simulink model "APSA"  (R2014b)
settings: Solver=FixedStepDiscrete  StartTime=0.0  StopTime=180  FixedStep=0.01  RelTol=1e-3
PreLoadFcn:
  | if exist('tl_preloadfcn','file'), tl_preloadfcn(gcs,400); end
PostLoadFcn:
  | if exist('tl_postloadfcn','file'), tl_postloadfcn(gcs,400); end
InitFcn:
  | if exist('tlds_init','file'), tlds_init(gcs); end
StartFcn:
  | if exist('tlds_start','file'), tlds_start(gcs); end
StopFcn:
  | if exist('tlds_stop','file'), tlds_stop(gcs); end
values from neighbouring files (symbols this model uses):
  EERAM_Map_Backward_Values = EERAM_Current_Map_Backward.signals.values(row,:)    [Create_Map.m]    (also in EERAM_Map_Backward_Values_2.mat = [0 0 0 0 0 0 150 150 150 150 150 150 ... (100 elements, 1x10)
  EERAM_Map_Forward_Values = EERAM_Current_Map_Forward.signals.values(row,:)    [Create_Map.m]    (also in EERAM_Map_Forward_Values_2.mat = [150 150 150 150 150 150 150 150 150 150 150 150 ... (100 el)
undefined symbols (not defined in the file or in its folder): sigbuilder_block
libraries: tllib x2
(part 3 of 3)

== stateflow chart APSA/Subsystem/APSA/APSA_chart ==
  state Init [function]
    (default) -> (junction 81) : {Index_vector = 0;
        | Counter_Time = 0;
        | Segments_Cnt = 0;
        | Cnt_Fail_Sens_Current = 0;
        | EERAM_Current_Map_Forward_Write = EERAM_Current_Map_Forward_Read;
        | EERAM_Current_Map_Backward_Write = EERAM_Current_Map_Backward_Read;}
  state Check_Min_Threshold [function]
    (default) -> (junction 206)
    (junction 206) -> (junction 207) [order 2] : [ Cnt_Fail_Sens_Current != 0 ]
    (junction 206) -> (junction 205) [order 1] : [ Current <=  MIN_CURRENT_THRESHOLD ]
    (junction 205) -> (junction 209) [order 1] : [ Cnt_Fail_Sens_Current > MAX_CNT_MIN_CURRENT_THRESHOLD ]
    (junction 207) -> (junction 211) : { Cnt_Fail_Sens_Current--; }
    (junction 206) -> (junction 208) [order 3] : { Fail_Sens_Current = APSA_FALSE;}
    (junction 205) -> (junction 210) [order 2] : { Cnt_Fail_Sens_Current++; }
    (junction 209) -> (junction 212) : { Fail_Sens_Current = APSA_TRUE; }
    (junction 211) -> (junction 208)
    (junction 210) -> (junction 208)
    (junction 212) -> (junction 210)
    (junction 208) -> (junction 213)
  state SetTimer_Delay [function]
    (default) -> (junction 1476)
    (junction 1476) -> (junction 1477) [order 1] : [APSA_Delay >1]
        | {APSA_Delay --;}
    (junction 1476) -> (junction 1478) [order 2]
    (junction 1477) -> (junction 1479)
    (junction 1478) -> (junction 1479)
  state Calculate_Lenght_Segment [function]
    (default) -> (junction 360) : {Mod=(Lenght_Motor_Stroke)%%MAX_NUM_ELEMENT;}
    (junction 360) -> (junction 361) [order 1] : [Mod == 0]
    (junction 360) -> (junction 371) [order 2] : {Lenght_Segment=((Lenght_Motor_Stroke/MAX_NUM_ELEMENT)+1);}
    (junction 361) -> (junction 365) : {Lenght_Segment = Lenght_Motor_Stroke/MAX_NUM_ELEMENT;}
    (junction 365) -> (junction 371)
    (junction 371) -> (junction 374)
  state ANTIPINCH_ACTIVE_FORWARD
    en:
    Counter_Time = 0;
    //ex: EERAM_Current_Map_Forward_Write = EERAM_Current_Map_Forward_Write - (Average_Difference);
    state WAIT_INRUSH_TIME_FORWARD
      WAIT_INRUSH_TIME_FORWARD -> (junction 87) [order 1]
      (junction 87) -> (junction 88) [order 1] : [Counter_Time < INRUSH_TIME]
          | {Counter_Time ++;}
      (junction 87) -> (junction 90) [order 2]
      (junction 88) -> (junction 93)
      (junction 93) -> (junction 797) [order 1] : [Counter_Time == INRUSH_TIME -1]
          | {Reset_Filter = 1;}
      (junction 93) -> (junction 795) [order 2] : {Reset_Filter = 0;}
      (junction 797) -> (junction 799)
      (junction 795) -> (junction 90)
      (junction 799) -> (junction 795)
      (junction 90) -> (junction 96)
      (junction 96) -> (junction 832) [order 1] : [Current_Peak <= Current]
          | {Current_Peak = Current;}
      (junction 96) -> (junction 830) [order 2]
      (junction 832) -> (junction 834)
      (junction 834) -> (junction 830)
    state Antipinch_Active
    state WAIT_ADAPTATION_TIME_FORWARD
      en:
      Average_Current = 0;
      Average_EERAM_Current_Map = 0;
      Average_Difference = 0;
      Segments_Cnt = 0;
      Index_vector = Hall_Counter_Forward / Lenght_Segment;
      WAIT_ADAPTATION_TIME_FORWARD -> (junction 99) [order 1]
      (junction 99) -> (junction 100) [order 1] : [Counter_Time < ADAPTATION_TIME]
          | {Counter_Time++;
          | Average_Current += Current;}
      (junction 99) -> (junction 101) [order 2]
      (junction 100) -> (junction 127)
      (junction 127) -> (junction 128) [order 1] : [Hall_Counter_Forward >= ((Index_vector * Lenght_Segment) + Lenght_Segment) ...
          | && (Index_vector <= (MAX_NUM_ELEMENT-1))]
      (junction 127) -> (junction 102) [order 2]
      (junction 128) -> (junction 130) : {//Average_Current += Current;
          | //EERAM_Current_Map_Forward_Write[Index_vector] = Map_Realignment(EERAM_Current_Map_Forward_Read[Index_vector],EERAM_Threshold_Attention_Higher);
          | Average_EERAM_Current_Map += EERAM_Current_Map_Forward_Read[Index_vector];
          | Index_vector++;
          | Segments_Cnt++;}
      (junction 102) -> (junction 101)
      (junction 130) -> (junction 102)
    state CHECK_ANTIPINCH_FORWARD
      en:
      cnt_antipinch = 0;
      Index_vector = Hall_Counter_Forward / Lenght_Segment;
      Current_Read = Current;
      Counter_Sample_Current = 1;
      APSA_Delay = 0;
      Cmd_Motor_Lift_Old = Cmd_Motor_Lift;
      state CounterManagerUpFwd(ResetCounter) [function]
        (default) -> (junction 1125) : {BitMaskIndex = (Index_vector / 8) ;
            | BitPosition = Index_vector - (BitMaskIndex * 8);
            | BitPosition = ((8 - BitPosition)*2 ) -2  ;}
        (junction 1125) -> (junction 1127) [order 1] : [ResetCounter == APSA_TRUE]
            | {CounterVectorUpFwd_Write[BitMaskIndex] = 0;
            | CounterVectorUpFwd_Write[BitMaskIndex] = 0;}
        (junction 1125) -> (junction 1083) [order 2]
        (junction 1127) -> (junction 1082)
        (junction 1083) -> (junction 1082) [commented out] : /*Counter = 4*/
            | [((CounterVectorFwd[BitMaskIndex] & (COUNT_BIT_TWO << (BitPosition))) ==  COUNT_BIT_TWO  << (BitPosition) ) ...
            | && ((CounterVectorFwd[BitMaskIndex] & (COUNT_BIT_ONE << (BitPosition))) ==  COUNT_BIT_ONE  << (BitPosition) )]
            | {CounterVectorFwd[BitMaskIndex] = (CounterVectorFwd[BitMaskIndex] & ~(COUNT_BIT_ONE << (BitPosition) ));
            | CounterVectorFwd[BitMaskIndex] = (CounterVectorFwd[BitMaskIndex] & ~(COUNT_BIT_TWO << (BitPosition)) );}
        (junction 1082) -> (junction 1085)
        (junction 1083) -> (junction 1084)
        (junction 1084) -> (junction 1085) [order 1] : [((CounterVectorUpFwd_Read[BitMaskIndex] & ((COUNT_BIT_TWO << (BitPosition)))) ==  COUNT_BIT_TWO  << (BitPosition) )]
            | /*{CounterVectorUpFwd_Write[BitMaskIndex] = (CounterVectorUpFwd_Read[BitMaskIndex] | COUNT_BIT_TWO << (BitPosition) );
            | CounterVectorUpFwd_Write[BitMaskIndex] = (CounterVectorUpFwd_Read[BitMaskIndex] | COUNT_BIT_ONE << (BitPosition) );}*/
            | {CounterVectorUpFwd_Write[BitMaskIndex] = (CounterVectorUpFwd_Read[BitMaskIndex] & ~(COUNT_BIT_ONE << (BitPosition) ));
            | CounterVectorUpFwd_Write[BitMaskIndex] = (CounterVectorUpFwd_Read[BitMaskIndex] & ~(COUNT_BIT_TWO << (BitPosition)) );
            | UpdateTrh = APSA_TRUE;}
        (junction 1084) -> (junction 1086) [order 2]
        (junction 1085) -> (junction 1087)
        (junction 1086) -> (junction 1087) [order 1] : [(CounterVectorUpFwd_Read[BitMaskIndex] & (COUNT_BIT_ONE << (BitPosition)))  == (COUNT_BIT_ONE << (BitPosition))  ]
            | {CounterVectorUpFwd_Write[BitMaskIndex] = (CounterVectorUpFwd_Read[BitMaskIndex] & ~(COUNT_BIT_ONE << (BitPosition)));
            | CounterVectorUpFwd_Write[BitMaskIndex] = (CounterVectorUpFwd_Read[BitMaskIndex] | (COUNT_BIT_TWO << (BitPosition)));}
        (junction 1087) -> (junction 1089)
        (junction 1086) -> (junction 1088) [order 2]
        (junction 1088) -> (junction 1089) : /*[(CounterVectorFwd[BitMaskIndex]  & (COUNT_BIT_ONE << ( BitPosition))) != (COUNT_BIT_ONE << BitPosition)]*/
            | {CounterVectorUpFwd_Write[BitMaskIndex] = (CounterVectorUpFwd_Read[BitMaskIndex] | (COUNT_BIT_ONE << (BitPosition) ));}
        (junction 1088) -> (junction 1090) [commented out]
        (junction 1089) -> (junction 1091) [commented out]
        (junction 1090) -> (junction 1091) [commented out] : {CounterVectorFwd[BitMaskIndex] = (CounterVectorFwd[BitMaskIndex] & ~COUNT_BIT_ONE << (BitPosition) );
            | CounterVectorFwd[BitMaskIndex] = (CounterVectorFwd[BitMaskIndex] & ~COUNT_BIT_TWO << (BitPosition) );}
      state CounterManagerDownFwd(ResetCounter) [function]
        (default) -> (junction 1133) : {BitMaskIndex = Index_vector / 8;
            | BitPosition = Index_vector - (BitMaskIndex * 8);
            | BitPosition = ((8 - BitPosition)*2 ) -2  ;}
        (junction 1133) -> (junction 1134) [order 1] : [ResetCounter == APSA_TRUE]
            | {CounterVectorDownFwd_Write[BitMaskIndex] = 0;
            | CounterVectorDownFwd_Write[BitMaskIndex] = 0;}
        (junction 1133) -> (junction 1136) [order 2]
        (junction 1134) -> (junction 1135)
        (junction 1136) -> (junction 1135) [commented out] : /*Counter = 4*/
            | [((CounterVectorFwd[BitMaskIndex] & (COUNT_BIT_TWO << (BitPosition))) ==  COUNT_BIT_TWO  << (BitPosition) ) ...
            | && ((CounterVectorFwd[BitMaskIndex] & (COUNT_BIT_ONE << (BitPosition))) ==  COUNT_BIT_ONE  << (BitPosition) )]
            | {CounterVectorFwd[BitMaskIndex] = (CounterVectorFwd[BitMaskIndex] & ~(COUNT_BIT_ONE << (BitPosition) ));
            | CounterVectorFwd[BitMaskIndex] = (CounterVectorFwd[BitMaskIndex] & ~(COUNT_BIT_TWO << (BitPosition)) );}
        (junction 1135) -> (junction 1138)
        (junction 1136) -> (junction 1137)
        (junction 1137) -> (junction 1138) [order 1] : [((CounterVectorDownFwd_Read[BitMaskIndex] & ((COUNT_BIT_TWO << (BitPosition)))) ==  COUNT_BIT_TWO  << (BitPosition) )]
            | /*{CounterVectorDownFwd_Write[BitMaskIndex] = (CounterVectorFwd_Read[BitMaskIndex] | COUNT_BIT_TWO << (BitPosition) );
            | CounterVectorDownFwd_Write[BitMaskIndex] = (CounterVectorFwd_Read[BitMaskIndex] | COUNT_BIT_ONE << (BitPosition) );}*/
            | {CounterVectorDownFwd_Write[BitMaskIndex] = (CounterVectorDownFwd_Read[BitMaskIndex] & ~(COUNT_BIT_ONE << (BitPosition) ));
            | CounterVectorDownFwd_Write[BitMaskIndex] = (CounterVectorDownFwd_Read[BitMaskIndex] & ~(COUNT_BIT_TWO << (BitPosition)) );
            | UpdateTrh = APSA_TRUE;}
        (junction 1137) -> (junction 1139) [order 2]
        (junction 1138) -> (junction 1140)
        (junction 1139) -> (junction 1140) [order 1] : [(CounterVectorDownFwd_Read[BitMaskIndex] & (COUNT_BIT_ONE << (BitPosition)))  == (COUNT_BIT_ONE << (BitPosition))  ]
            | {CounterVectorDownFwd_Write[BitMaskIndex] = (CounterVectorDownFwd_Read[BitMaskIndex] & ~(COUNT_BIT_ONE << (BitPosition)));
            | CounterVectorDownFwd_Write[BitMaskIndex] = (CounterVectorDownFwd_Read[BitMaskIndex] | (COUNT_BIT_TWO << (BitPosition)));}
        (junction 1140) -> (junction 1142)
        (junction 1139) -> (junction 1141) [order 2]
        (junction 1141) -> (junction 1142) : /*[(CounterVectorFwd[BitMaskIndex]  & (COUNT_BIT_ONE << ( BitPosition))) != (COUNT_BIT_ONE << BitPosition)]*/
            | {CounterVectorDownFwd_Write[BitMaskIndex] = (CounterVectorDownFwd_Read[BitMaskIndex] | (COUNT_BIT_ONE << (BitPosition) ));}
        (junction 1141) -> (junction 1143) [commented out]
        (junction 1142) -> (junction 1144) [commented out]
        (junction 1143) -> (junction 1144) [commented out] : {CounterVectorFwd[BitMaskIndex] = (CounterVectorFwd[BitMaskIndex] & ~COUNT_BIT_ONE << (BitPosition) );
            | CounterVectorFwd[BitMaskIndex] = (CounterVectorFwd[BitMaskIndex] & ~COUNT_BIT_TWO << (BitPosition) );}
      CHECK_ANTIPINCH_FORWARD -> (junction 275) [order 1] : {SetTimer_Delay();}
      (junction 275) -> (junction 891) [order 2]
      (junction 891) -> (junction 1491) [order 1] : [ Hall_Counter_Forward >= ((Index_vector * Lenght_Segment) + Lenght_Segment) ...
          | && (Index_vector < (MAX_NUM_ELEMENT - 1))]
      (junction 1491) -> (junction 1488) [order 2]
      (junction 1488) -> (junction 1497) [order 1] : /* with voltage drop  || stop lift motor inhibit antipinch for DROP_DELAY */
          | [(((Vbatt_Old - Vbatt) >= VBATT_DROP) || ((Vbatt - Vbatt_Old) >= VBATT_DROP)) ...
          | || ((Cmd_Motor_Lift == APSA_CMD_STOP) && ((Cmd_Motor_Lift_Old == APSA_CMD_FORWARD) || (Cmd_Motor_Lift_Old == APSA_CMD_BACKWARD)))]
          | {APSA_Delay = DROP_DELAY;}
      (junction 275) -> (junction 706) [order 1] : [cnt_antipinch >T_ANTIPINCH]
      (junction 891) -> (junction 282) [order 2] : {Current_Read += Current;
          | Counter_Sample_Current ++;}
      (junction 1491) -> (junction 1500) [order 1] : /*this check is used to avoid currentread saturation
          | during drop delay*/
          | [APSA_Delay > 1]
      (junction 1488) -> (junction 1494) [order 2] : {Current_Read_Average = Current_Read / Counter_Sample_Current;
          |  Delta_Current_actual = ( Current_Read_Average - (EERAM_Current_Map_Forward_Read[Index_vector] + Average_Difference ) - Delta_Current_previuos );}
      (junction 1497) -> (junction 1496)
      (junction 1494) -> (junction 1496) [order 1] : [APSA_Delay ==  1]
          | {Delta_Current_previuos  += Delta_Current_actual;
          | APSA_Delay = 0; }
      (junction 1494) -> (junction 280) [order 2]
      (junction 1496) -> (junction 1108)
      (junction 280) -> (junction 883) [order 2] : {cnt_antipinch = 0;
          | UpdateTrh = APSA_FALSE;}
      (junction 280) -> (junction 329) [order 1] : [(Delta_Current_actual  > Threshold_AntiPinch_Update) ...
          | && (cnt_antipinch < T_ANTIPINCH)  ]
          | {cnt_antipinch++; }
      (junction 883) -> (junction 299) : /*CHECK_ATTENTION_THRESHOLD*/
      (junction 299) -> (junction 302) [order 1] : /*UPPER_THRESHOLD*/
          | [Delta_Current_actual > Threshold_Attention_Update ]
          | {CounterManagerUpFwd(APSA_FALSE);
          | Delta_Current_previuos  += Threshold_Attention_Update;}
      (junction 302) -> (junction 1108) [order 1] : [UpdateTrh == APSA_TRUE]
          | {EERAM_Current_Map_Forward_Write[Index_vector] += (Delta_Current_actual / DELTA_1);}
      (junction 299) -> (junction 304) [order 2] : /*Reset counter Up*/
          | {CounterManagerUpFwd(APSA_TRUE); }
      (junction 302) -> (junction 1109) [order 2]
      (junction 1108) -> (junction 1299)
      (junction 1109) -> (junction 1299)
      (junction 1299) -> (junction 1106)
      (junction 304) -> (junction 306) [order 1] : /*LOWER_THRESHOLD*/
          | [Delta_Current_actual < (-Threshold_Attention_Update) ...
          | && EERAM_Current_Map_Forward_Read[Index_vector] > MIN_CURRENT_THRESHOLD ]
          | {CounterManagerDownFwd(APSA_FALSE);
          | Delta_Current_previuos  += Delta_Current_actual;}
      (junction 306) -> (junction 1106) [order 1] : [UpdateTrh == APSA_TRUE]
          | {EERAM_Current_Map_Forward_Write[Index_vector]-= (-Delta_Current_actual / DELTA_2 );}
      (junction 329) -> (junction 331) [order 1] : [cnt_antipinch >= T_ANTIPINCH]
          | {Antipinch_Active = APSA_ACTIVE;}
      (junction 304) -> (junction 885) [order 2] : /*Reset counter Down*/
          | {CounterManagerDownFwd(APSA_TRUE);
          | Delta_Current_previuos  += Delta_Current_actual;}
      (junction 306) -> (junction 887) [order 2]
      (junction 1106) -> (junction 1115)
      (junction 329) -> (junction 333) [order 2]
      (junction 331) -> (junction 335)
      (junction 1500) -> (junction 333)
      (junction 335) -> (junction 333)
      (junction 885) -> (junction 335)
      (junction 887) -> (junction 885)
      (junction 1115) -> (junction 887)
      (junction 333) -> (junction 338) : {Check_Min_Threshold();
          | Index_vector++;
          | Current_Read = Current;
          | Counter_Sample_Current = 1;
          | Vbatt_Old = Vbatt;
          | Cmd_Motor_Lift_Old = Cmd_Motor_Lift; }
      (junction 706) -> (junction 282)
      (junction 282) -> (junction 338)
      (junction 338) -> (junction 346)
    (default) -> WAIT_INRUSH_TIME_FORWARD : {Current_Peak = Current;}
    WAIT_INRUSH_TIME_FORWARD -> (junction 875) [order 1] : [Counter_Time >= INRUSH_TIME]
        | {Counter_Time = 0;}
    (junction 875) -> ANTIPINCH_ACTIVE_FORWARD.Antipinch_Active [commented out] : [Current  > (Current_Peak - DELTA_PEACK)]
        | {Antipinch_Active = APSA_ACTIVE;}
    (junction 875) -> WAIT_ADAPTATION_TIME_FORWARD
    (junction 857) -> ANTIPINCH_ACTIVE_FORWARD.Antipinch_Active
    WAIT_ADAPTATION_TIME_FORWARD -> CHECK_ANTIPINCH_FORWARD [order 1] : [Counter_Time >= ADAPTATION_TIME]
        | {Average_Current /= Counter_Time;
        | Average_EERAM_Current_Map /= Segments_Cnt;
        | Average_Difference  = Average_Current - Average_EERAM_Current_Map ;
        | //EERAM_Current_Map_Forward_Write = EERAM_Current_Map_Forward_Write + (Average_Difference);
        | Delta_Current_previuos = 0;
        | Threshold_Attention_Update = EERAM_Threshold_Antipinch_Forward / 2;
        | Threshold_AntiPinch_Update = EERAM_Threshold_Antipinch_Forward ;}
    CHECK_ANTIPINCH_FORWARD -> (junction 857) [order 1] : [Antipinch_Active == APSA_ACTIVE]
        | {Current_Read_Average = 0;}
  state IDLE
    en:
    Antipinch_Active = APSA_NOT_ACTIVE;
  state WRITE_MAP_FORWARD
    en:
    Index_vector = Hall_Counter_Forward / Lenght_Segment;
    //Current_Read = Current;
    Current_Read = 0;
    Counter_Sample_Current = 1;
    Index_peak_time = 0;
    Counter_Time = 0;
    WRITE_MAP_FORWARD -> (junction 1371) [order 1]
    (junction 1371) -> (junction 1368) [order 1] : [Counter_Time < PEAK_FILTER_TIME]
        | {Counter_Time++;}
    (junction 1368) -> (junction 1366) [order 1] : [Hall_Counter_Forward >= ((Index_vector * Lenght_Segment) + Lenght_Segment) ...
        | && (Index_vector <= (MAX_NUM_ELEMENT-1))]
        | {Index_vector++;}
    (junction 1371) -> (junction 1369) [order 2] : //[Counter_Time >= PEAK_FILTER_TIME]
    (junction 1368) -> (junction 1366) [order 2]
    (junction 1366) -> (junction 1381)
    (junction 1381) -> (junction 1383)
    (junction 1369) -> (junction 1370) [order 1] : /*Thi for cycle is used to erase the hit of the current */
        | [Index_peak_time <= Index_vector]
    (junction 1370) -> (junction 1367) : {EERAM_Current_Map_Forward_Write[Index_peak_time] = Current;
        | Index_peak_time ++;}
    (junction 1367) -> (junction 1369)
    (junction 1369) -> (junction 1392) [order 2]
    (junction 1392) -> (junction 63) [order 2]
    (junction 1392) -> (junction 63) [order 1] : [Current_Read == 0]
        | {Current_Read = Current;}
    (junction 63) -> (junction 64) [order 1] : [Hall_Counter_Forward >= ((Index_vector * Lenght_Segment) + Lenght_Segment) ...
        | && (Index_vector <= (MAX_NUM_ELEMENT-1))]
    (junction 64) -> (junction 730) [order 1] : [Counter_Sample_Current == 0 ...
        | || Current_Read == 0 ]
    (junction 63) -> (junction 66) [order 2] : {Current_Read += Current;
        | Counter_Sample_Current++;}
    (junction 64) -> (junction 734) [order 2] : {Current_Read_Average = Current_Read / Counter_Sample_Current;}
    (junction 730) -> (junction 732) : {Current_Read_Average = Current;}
    (junction 732) -> (junction 734)
    (junction 734) -> (junction 66) : {EERAM_Current_Map_Forward_Write[Index_vector] = Current_Read_Average;
        | Check_Min_Threshold();
        | Current_Read=Current;
        | Counter_Sample_Current = 1;
        | Index_vector++;}
    (junction 66) -> (junction 717)
    (junction 1383) -> (junction 717)
  state WRITE_MAP_BACKWARD
    en:
    Index_vector = Hall_Counter_Backward / Lenght_Segment;
    // Current_Read = Current;
    Current_Read = 0;
    Counter_Sample_Current = 1;
    Counter_Time = 0;
    Index_peak_time = 0;
    WRITE_MAP_BACKWARD -> (junction 1342) [order 1]
    (junction 1342) -> (junction 1340) [order 1] : [Counter_Time < PEAK_FILTER_TIME]
        | {Counter_Time++;}
    (junction 1340) -> (junction 1343) [order 1] : [ (Hall_Counter_Backward >= ((Index_vector * Lenght_Segment) + Lenght_Segment)) ...
        | && (Index_vector <= (MAX_NUM_ELEMENT-1))]
        | {Index_vector++;}
    (junction 1340) -> (junction 1343) [order 2]
    (junction 1342) -> (junction 1322) [order 2] : //[Counter_Time >= PEAK_FILTER_TIME]
    (junction 1343) -> (junction 1386)
    (junction 1386) -> (junction 1388)
    (junction 1322) -> (junction 1325) [order 1] : [Index_peak_time <= Index_vector]
    (junction 1325) -> (junction 1326) : {EERAM_Current_Map_Backward_Write[Index_peak_time] = Current;
        | Index_peak_time ++;}
    (junction 1326) -> (junction 1322)
    (junction 1322) -> (junction 1397) [order 2]
    (junction 1397) -> (junction 633) [order 2]
    (junction 1397) -> (junction 633) [order 1] : [Current_Read == 0]
        | {Current_Read = Current;}
    (junction 633) -> (junction 639) [order 1] : [ (Hall_Counter_Backward >= ((Index_vector * Lenght_Segment) + Lenght_Segment)) ...
        | && (Index_vector <= (MAX_NUM_ELEMENT-1))]
    (junction 639) -> (junction 739) [order 1] : [Counter_Sample_Current == 0 ...
        | || Current_Read == 0 ]
    (junction 633) -> (junction 632) [order 2] : {Current_Read += Current;
        | Counter_Sample_Current++;}
    (junction 639) -> (junction 641) [order 2] : {Current_Read_Average = Current_Read / Counter_Sample_Current;}
    (junction 739) -> (junction 741) : {Current_Read_Average =Current;}
    (junction 641) -> (junction 632) : {EERAM_Current_Map_Backward_Write[Index_vector]=Current_Read_Average;
        | Check_Min_Threshold();
        | Current_Read = Current;
        | Counter_Sample_Current = 1;
        | Index_vector++;}
    (junction 741) -> (junction 641)
    (junction 632) -> (junction 635)
    (junction 1388) -> (junction 635)
  state ANTIPINCH_ACTIVE_BACKWARD
    en:
    Counter_Time = 0;
    //ex: EERAM_Current_Map_Backward_Write = EERAM_Current_Map_Backward_Write - (Average_Difference);
    state WAIT_INRUSH_TIME_BACKWARD
      WAIT_INRUSH_TIME_BACKWARD -> (junction 803) [order 1]
      (junction 803) -> (junction 804) [order 1] : [Counter_Time < INRUSH_TIME]
          | {Counter_Time ++;}
      (junction 803) -> (junction 811) [order 2]
      (junction 804) -> (junction 807)
      (junction 807) -> (junction 817) [order 1] : [Counter_Time == INRUSH_TIME -1]
          | {Reset_Filter = 1;}
      (junction 807) -> (junction 813) [order 2] : {Reset_Filter = 0;}
      (junction 817) -> (junction 814)
      (junction 813) -> (junction 811)
      (junction 814) -> (junction 813)
      (junction 811) -> (junction 866)
      (junction 866) -> (junction 870) [order 1] : [Current_Peak <= Current]
          | {Current_Peak = Current;}
      (junction 866) -> (junction 869) [order 2]
      (junction 870) -> (junction 872)
      (junction 872) -> (junction 869)
    state Antipinch_Active
    state WAIT_ADAPTATION_TIME_BACKWARD
      en:
      Average_Current = 0;
      Average_EERAM_Current_Map = 0;
      Average_Difference = 0;
      Segments_Cnt = 0;
      Index_vector=Hall_Counter_Backward/Lenght_Segment;
      WAIT_ADAPTATION_TIME_BACKWARD -> (junction 656) [order 1]
      (junction 656) -> (junction 651) [order 1] : [Counter_Time < ADAPTATION_TIME]
          | {Counter_Time++;
          | Average_Current += Current;}
      (junction 656) -> (junction 652) [order 2]
      (junction 651) -> (junction 645)
      (junction 645) -> (junction 647) [order 1] : [Hall_Counter_Backward >= ((Index_vector * Lenght_Segment) + Lenght_Segment) ...
          | && (Index_vector <= (MAX_NUM_ELEMENT - 1))]
      (junction 645) -> (junction 654) [order 2]
      (junction 647) -> (junction 655) : {//Current_Read_Average = Current;
          | //Current_Read_Average = Current_Read / Counter_Sample_Current;
          | //Average_Current += Current_Read_Average;
          | //EERAM_Current_Map_Backward_Write[Index_vector]=Map_Realignment(EERAM_Current_Map_Backward_Read[Index_vector],EERAM_Threshold_Attention_Lower);
          | Average_EERAM_Current_Map += EERAM_Current_Map_Backward_Read[Index_vector];
          | Index_vector++;
          | Segments_Cnt++;}
      (junction 654) -> (junction 652)
      (junction 655) -> (junction 654)
    state CHECK_ANTIPINCH_BACKWARD
      en:
      cnt_antipinch = 0;
      Index_vector = Hall_Counter_Backward / Lenght_Segment;
      Current_Read = Current;
      Counter_Sample_Current = 1;
      Vbatt_Old = Vbatt;
      APSA_Delay = 0;
      Cmd_Motor_Lift_Old = Cmd_Motor_Lift;
      state CounterManagerDownBwd(ResetCounter) [function]
        (default) -> (junction 1257) : {BitMaskIndex = Index_vector / 8;
            | BitPosition = Index_vector - (BitMaskIndex * 8);
            | BitPosition = ((8 - BitPosition)*2 ) -2  ;}
        (junction 1257) -> (junction 1258) [order 1] : [ResetCounter == APSA_TRUE]
            | {CounterVectorDownBwd_Write[BitMaskIndex] = 0;
            | CounterVectorDownBwd_Write[BitMaskIndex] = 0;}
        (junction 1257) -> (junction 1260) [order 2]
        (junction 1258) -> (junction 1259)
        (junction 1260) -> (junction 1259) [commented out] : /*Counter = 4*/
            | [((CounterVectorBwd[BitMaskIndex] & (COUNT_BIT_TWO << (BitPosition))) ==  COUNT_BIT_TWO  << (BitPosition) ) ...
            | && ((CounterVectorBwd[BitMaskIndex] & (COUNT_BIT_ONE << (BitPosition))) ==  COUNT_BIT_ONE  << (BitPosition) )]
            | {CounterVectorBwd[BitMaskIndex] = (CounterVectorBwd[BitMaskIndex] & ~(COUNT_BIT_ONE << (BitPosition) ));
            | CounterVectorBwd[BitMaskIndex] = (CounterVectorBwd[BitMaskIndex] & ~(COUNT_BIT_TWO << (BitPosition)) );}
        (junction 1259) -> (junction 1262)
        (junction 1260) -> (junction 1261)
        (junction 1261) -> (junction 1262) [order 1] : /*Counter = 3*/
            | [((CounterVectorDownBwd_Read[BitMaskIndex] & ((COUNT_BIT_TWO << (BitPosition)))) ==  COUNT_BIT_TWO  << (BitPosition) )]
            | /*{CounterVectorBwd[BitMaskIndex] = (CounterVectorBwd[BitMaskIndex] | COUNT_BIT_TWO << (BitPosition) );
            | CounterVectorBwd[BitMaskIndex] = (CounterVectorBwd[BitMaskIndex] | COUNT_BIT_ONE << (BitPosition) );}*/
            | {CounterVectorDownBwd_Write[BitMaskIndex] = (CounterVectorDownBwd_Read[BitMaskIndex] & ~(COUNT_BIT_ONE << (BitPosition) ));
            | CounterVectorDownBwd_Write[BitMaskIndex] = (CounterVectorDownBwd_Read[BitMaskIndex] & ~(COUNT_BIT_TWO << (BitPosition)) );
            | UpdateTrh = APSA_TRUE;}
        (junction 1261) -> (junction 1263) [order 2]
        (junction 1262) -> (junction 1264)
        (junction 1263) -> (junction 1264) [order 1] : /*Counter = 2*/
            | [(CounterVectorDownBwd_Read[BitMaskIndex] & (COUNT_BIT_ONE << (BitPosition)))  == (COUNT_BIT_ONE << (BitPosition))]
            | {CounterVectorDownBwd_Write[BitMaskIndex] = (CounterVectorDownBwd_Read[BitMaskIndex] & ~(COUNT_BIT_ONE << (BitPosition)));
            | CounterVectorDownBwd_Write[BitMaskIndex] = (CounterVectorDownBwd_Read[BitMaskIndex] | (COUNT_BIT_TWO << (BitPosition)));}
        (junction 1263) -> (junction 1265) [order 2]
        (junction 1264) -> (junction 1266)
        (junction 1265) -> (junction 1266) : /*Counter = 1*/
            | //[(CounterVectorBwd_Read[BitMaskIndex]  & (COUNT_BIT_ONE << ( BitPosition))) != (COUNT_BIT_ONE << BitPosition)]
            | {CounterVectorDownBwd_Write[BitMaskIndex] = (CounterVectorDownBwd_Read[BitMaskIndex] | (COUNT_BIT_ONE << (BitPosition) ));}
        (junction 1265) -> (junction 1267) [commented out]
        (junction 1266) -> (junction 1268) [commented out]
        (junction 1267) -> (junction 1268) [commented out] : {CounterVectorBwd[BitMaskIndex] = (CounterVectorBwd[BitMaskIndex] & ~COUNT_BIT_ONE << (BitPosition) );
            | CounterVectorBwd[BitMaskIndex] = (CounterVectorBwd[BitMaskIndex] & ~COUNT_BIT_TWO << (BitPosition) );}
      state CounterManagerUpBwd(ResetCounter) [function]
        (default) -> (junction 1249) : {BitMaskIndex = Index_vector / 8;
            | BitPosition = Index_vector - (BitMaskIndex * 8);
            | BitPosition = ((8 - BitPosition)*2 ) -2  ;}
        (junction 1249) -> (junction 1251) [order 1] : [ResetCounter == APSA_TRUE]
            | {CounterVectorUpBwd_Write[BitMaskIndex] = 0;
            | CounterVectorUpBwd_Write[BitMaskIndex] = 0;}
        (junction 1251) -> (junction 1039)
        (junction 1249) -> (junction 1042) [order 2]
        (junction 1042) -> (junction 1039) [commented out] : /*Counter = 4*/
            | [((CounterVectorBwd[BitMaskIndex] & (COUNT_BIT_TWO << (BitPosition))) ==  COUNT_BIT_TWO  << (BitPosition) ) ...
            | && ((CounterVectorBwd[BitMaskIndex] & (COUNT_BIT_ONE << (BitPosition))) ==  COUNT_BIT_ONE  << (BitPosition) )]
            | {CounterVectorBwd[BitMaskIndex] = (CounterVectorBwd[BitMaskIndex] & ~(COUNT_BIT_ONE << (BitPosition) ));
            | CounterVectorBwd[BitMaskIndex] = (CounterVectorBwd[BitMaskIndex] & ~(COUNT_BIT_TWO << (BitPosition)) );}
        (junction 1039) -> (junction 1032)
        (junction 1042) -> (junction 1037)
        (junction 1037) -> (junction 1032) [order 1] : /*Counter = 3*/
            | [((CounterVectorUpBwd_Read[BitMaskIndex] & ((COUNT_BIT_TWO << (BitPosition)))) ==  COUNT_BIT_TWO  << (BitPosition) )]
            | /*{CounterVectorBwd[BitMaskIndex] = (CounterVectorBwd[BitMaskIndex] | COUNT_BIT_TWO << (BitPosition) );
            | CounterVectorBwd[BitMaskIndex] = (CounterVectorBwd[BitMaskIndex] | COUNT_BIT_ONE << (BitPosition) );}*/
            | {CounterVectorUpBwd_Write[BitMaskIndex] = (CounterVectorUpBwd_Read[BitMaskIndex] & ~(COUNT_BIT_ONE << (BitPosition) ));
            | CounterVectorUpBwd_Write[BitMaskIndex] = (CounterVectorUpBwd_Read[BitMaskIndex] & ~(COUNT_BIT_TWO << (BitPosition)) );
            | UpdateTrh = APSA_TRUE;}
        (junction 1037) -> (junction 1036) [order 2]
        (junction 1032) -> (junction 1033)
        (junction 1036) -> (junction 1033) [order 1] : /*Counter = 2*/
            | [(CounterVectorUpBwd_Read[BitMaskIndex] & (COUNT_BIT_ONE << (BitPosition)))  == (COUNT_BIT_ONE << (BitPosition))]
            | {CounterVectorUpBwd_Write[BitMaskIndex] = (CounterVectorUpBwd_Read[BitMaskIndex] & ~(COUNT_BIT_ONE << (BitPosition)));
            | CounterVectorUpBwd_Write[BitMaskIndex] = (CounterVectorUpBwd_Read[BitMaskIndex] | (COUNT_BIT_TWO << (BitPosition)));}
        (junction 1033) -> (junction 1030)
        (junction 1036) -> (junction 1018) [order 2]
        (junction 1018) -> (junction 1030) : /*Counter = 1*/
            | //[(CounterVectorBwd_Read[BitMaskIndex]  & (COUNT_BIT_ONE << ( BitPosition))) != (COUNT_BIT_ONE << BitPosition)]
            | {CounterVectorUpBwd_Write[BitMaskIndex] = (CounterVectorUpBwd_Read[BitMaskIndex] | (COUNT_BIT_ONE << (BitPosition) ));}
        (junction 1018) -> (junction 1031) [commented out]
        (junction 1030) -> (junction 1029) [commented out]
        (junction 1031) -> (junction 1029) [commented out] : {CounterVectorBwd[BitMaskIndex] = (CounterVectorBwd[BitMaskIndex] & ~COUNT_BIT_ONE << (BitPosition) );
            | CounterVectorBwd[BitMaskIndex] = (CounterVectorBwd[BitMaskIndex] & ~COUNT_BIT_TWO << (BitPosition) );}
      CHECK_ANTIPINCH_BACKWARD -> (junction 899) [order 1] : {SetTimer_Delay();}
      (junction 899) -> (junction 903) [order 2]
      (junction 903) -> (junction 1468) [order 1] : /*End of segment */
          | [Hall_Counter_Backward >= ((Index_vector * Lenght_Segment) + Lenght_Segment) ...
          | && Index_vector < (MAX_NUM_ELEMENT-1) ]
      (junction 1468) -> (junction 1457) [order 2]
      (junction 1457) -> (junction 1399) [order 1] : /* with voltage drop  || stop lift motor inhibit antipinch for DROP_DELAY */
          | [(((Vbatt_Old - Vbatt) >= VBATT_DROP) || ((Vbatt - Vbatt_Old) >= VBATT_DROP)) ...
          | || ((Cmd_Motor_Lift == APSA_CMD_STOP) &&((Cmd_Motor_Lift_Old == APSA_CMD_FORWARD) || (Cmd_Motor_Lift_Old == APSA_CMD_BACKWARD)))]
          | {APSA_Delay = DROP_DELAY;}
      (junction 899) -> (junction 915) [order 1] : [cnt_antipinch >T_ANTIPINCH]
      (junction 903) -> (junction 913) [order 2] : {Current_Read += Current;
          | Counter_Sample_Current ++;}
      (junction 1468) -> (junction 1471) [order 1] : /*this check is used to avoid currentread saturation
          | during drop delay*/
          | [APSA_Delay > 1]
      (junction 1457) -> (junction 902) [order 2] : {Current_Read_Average = Current_Read / Counter_Sample_Current;
          | Delta_Current_actual = (Current_Read_Average - (EERAM_Current_Map_Backward_Read[Index_vector] + Average_Difference)  - Delta_Current_previuos );}
      (junction 1399) -> (junction 1462)
      (junction 902) -> (junction 1462) [order 1] : [APSA_Delay ==  1]
          | {Delta_Current_previuos  += Delta_Current_actual;
          | APSA_Delay = 0; }
      (junction 902) -> (junction 900) [order 2]
      (junction 1462) -> (junction 1070)
      (junction 900) -> (junction 905) [order 2] : {cnt_antipinch = 0;
          | UpdateTrh = APSA_FALSE;}
      (junction 900) -> (junction 908) [order 1] : [(Delta_Current_actual  > Threshold_AntiPinch_Update) ...
          | && (cnt_antipinch < T_ANTIPINCH)  ]
          | {cnt_antipinch++; }
      (junction 905) -> (junction 904) : /*CHECK_ATTENTION_THRESHOLD*/
      (junction 904) -> (junction 901) [order 1] : /*UPPER_THRESHOLD*/
          | [Delta_Current_actual > Threshold_Attention_Update ]
          | {CounterManagerUpBwd(APSA_FALSE);
          | Delta_Current_previuos  += Threshold_Attention_Update;}
      (junction 901) -> (junction 1070) [order 1] : [UpdateTrh == APSA_TRUE]
          | {EERAM_Current_Map_Backward_Write[Index_vector] += (Delta_Current_actual / DELTA_1);}
      (junction 904) -> (junction 906) [order 2] : {CounterManagerUpBwd(APSA_TRUE); }
      (junction 901) -> (junction 1068) [order 2]
      (junction 1070) -> (junction 1301)
      (junction 1068) -> (junction 1301)
      (junction 1301) -> (junction 1077)
      (junction 906) -> (junction 907) [order 1] : /*LOWER_THRESHOLD*/
          | [Delta_Current_actual < (-Threshold_Attention_Update) ...
          | && EERAM_Current_Map_Backward_Read[Index_vector] > MIN_CURRENT_THRESHOLD ]
          | {CounterManagerDownBwd(APSA_FALSE);
          | Delta_Current_previuos  += Delta_Current_actual; }
      (junction 907) -> (junction 1077) [order 1] : [UpdateTrh == APSA_TRUE]
          | {EERAM_Current_Map_Backward_Write[Index_vector] -= (-Delta_Current_actual / DELTA_2 );}
      (junction 906) -> (junction 911) [order 2] : {CounterManagerDownBwd(APSA_TRUE);
          | Delta_Current_previuos  += Delta_Current_actual; }
      (junction 907) -> (junction 912) [order 2]
      (junction 1077) -> (junction 1074)
      (junction 908) -> (junction 909) [order 1] : [cnt_antipinch >= T_ANTIPINCH]
          | {Antipinch_Active = APSA_ACTIVE;}
      (junction 908) -> (junction 910) [order 2]
      (junction 909) -> (junction 897)
      (junction 1471) -> (junction 910)
      (junction 897) -> (junction 910)
      (junction 911) -> (junction 897)
      (junction 912) -> (junction 911)
      (junction 1074) -> (junction 912)
      (junction 910) -> (junction 914) : {Check_Min_Threshold();
          | Index_vector++;
          | Current_Read = Current;
          | Counter_Sample_Current = 1;
          | Vbatt_Old = Vbatt;
          | Cmd_Motor_Lift_Old = Cmd_Motor_Lift; }
      (junction 915) -> (junction 913)
      (junction 913) -> (junction 914)
      (junction 914) -> (junction 898)
    (default) -> WAIT_INRUSH_TIME_BACKWARD : {Current_Peak = Current;}
    WAIT_INRUSH_TIME_BACKWARD -> (junction 877) [order 1] : [Counter_Time >= INRUSH_TIME]
        | {Counter_Time = 0;}
    (junction 877) -> ANTIPINCH_ACTIVE_BACKWARD.Antipinch_Active [commented out] : [Current  < (Current_Peak - DELTA_PEACK)]
        | {Antipinch_Active = APSA_ACTIVE;}
    (junction 877) -> WAIT_ADAPTATION_TIME_BACKWARD
    (junction 861) -> ANTIPINCH_ACTIVE_BACKWARD.Antipinch_Active
    WAIT_ADAPTATION_TIME_BACKWARD -> CHECK_ANTIPINCH_BACKWARD [order 1] : [Counter_Time >= ADAPTATION_TIME]
        | {Average_Current /= Counter_Time;
        | Average_EERAM_Current_Map /= Segments_Cnt;
        | Average_Difference  = Average_Current - Average_EERAM_Current_Map ;
        | //EERAM_Current_Map_Backward_Write = EERAM_Current_Map_Backward_Write + Average_Difference;
        | Delta_Current_previuos = 0;
        | Threshold_Attention_Update = EERAM_Threshold_Antipinch_Backward / 2 ;
        | Threshold_AntiPinch_Update = EERAM_Threshold_Antipinch_Backward ;}
    CHECK_ANTIPINCH_BACKWARD -> (junction 861) [order 1] : [Antipinch_Active == APSA_ACTIVE]
        | {Current_Read_Average = 0;}
  (default) -> IDLE : {Init();
      | Calculate_Lenght_Segment();}
  ANTIPINCH_ACTIVE_FORWARD -> IDLE [order 1] : [Check_Antipinch == APSA_NOT_ACTIVE]
  IDLE -> WRITE_MAP_FORWARD [order 3] : [Write_Map ==  APSA_ACTIVE...
      | && Cmd_Motor ==APSA_CMD_FORWARD...
      | && Enable_APSA == APSA_ACTIVE]
      | {EERAM_Current_Map_Forward_Write = 0;}
  IDLE -> ANTIPINCH_ACTIVE_FORWARD [order 2] : [Check_Antipinch == APSA_ACTIVE...
      | && Cmd_Motor == APSA_CMD_FORWARD...
      | && Enable_APSA == APSA_ACTIVE]
  WRITE_MAP_FORWARD -> IDLE [order 1] : [Write_Map ==  APSA_NOT_ACTIVE]
  ANTIPINCH_ACTIVE_BACKWARD -> ANTIPINCH_ACTIVE_FORWARD [order 2] : [Check_Antipinch == APSA_ACTIVE...
      | && Cmd_Motor == APSA_CMD_FORWARD]
  ANTIPINCH_ACTIVE_FORWARD -> ANTIPINCH_ACTIVE_BACKWARD [order 2] : [Check_Antipinch == APSA_ACTIVE...
      | && Cmd_Motor== APSA_CMD_BACKWARD]
  WRITE_MAP_BACKWARD -> WRITE_MAP_FORWARD [order 2] : [Write_Map == APSA_ACTIVE...
      | && Cmd_Motor==APSA_CMD_FORWARD]
      | {EERAM_Current_Map_Forward_Write=0;}
  WRITE_MAP_FORWARD -> WRITE_MAP_BACKWARD [order 2] : [Write_Map == APSA_ACTIVE...
      | && Cmd_Motor==APSA_CMD_BACKWARD]
      | {EERAM_Current_Map_Backward_Write=0;}
  IDLE -> WRITE_MAP_BACKWARD [order 1] : [Write_Map ==  APSA_ACTIVE...
      | && Cmd_Motor==APSA_CMD_BACKWARD...
      | && Enable_APSA == APSA_ACTIVE]
      | {Calculate_Lenght_Segment();
      | EERAM_Current_Map_Backward_Write=0;}
  ANTIPINCH_ACTIVE_BACKWARD -> IDLE [order 1] : [Check_Antipinch == APSA_NOT_ACTIVE]
  IDLE -> ANTIPINCH_ACTIVE_BACKWARD [order 4] : [Check_Antipinch == APSA_ACTIVE...
      | && Cmd_Motor==APSA_CMD_BACKWARD...
      | &&Enable_APSA == APSA_ACTIVE]
  WRITE_MAP_BACKWARD -> IDLE [order 1] : [Write_Map ==  APSA_NOT_ACTIVE]
  data: ResetCounter function_input uint8; ResetCounter function_input uint8; ResetCounter function_input uint8; ResetCounter function_input uint8; EERAM_Current_Map_Forward_Read input int16 size=100; EERAM_Current_Map_Backward_Read input int16 size=100; EERAM_Threshold_Attention_Forward input uint8; EERAM_Threshold_Attention_Backward input uint8; EERAM_Threshold_Antipinch_Forward input uint8; EERAM_Threshold_Antipinch_Backward input uint8; Check_Antipinch input uint8; Cmd_Motor input uint8; Write_Map input uint8; Lenght_Motor_Stroke input uint16; Cmd_Motor_Lift input uint8; Hall_Counter_Forward input int16; Hall_Counter_Backward input int16; Current input int16; Enable_APSA input uint8; Vbatt input uint16; Lenght_Segment local uint8; EERAM_Current_Map_Forward_Write output int16 size=100; EERAM_Current_Map_Backward_Write output int16 size=100; Counter_Time local uint16; Average_EERAM_Current_Map local int16; Average_Current local int16; Mod local uint8; Segments_Cnt local uint8 [..100]; Average_Difference local int16; Fail_Sens_Current output uint8; Cnt_Fail_Sens_Current local uint8; cnt_antipinch output uint16; DELTA_1 input uint8; DELTA_2 input uint8; DELTA_3 input uint8; DELTA_4 input uint8; Antipinch_Active output uint8; DELTA_5 input uint8; DELTA_6 input uint8; Index_vector output uint8; Threshold_AntiPinch_Update output int16; Threshold_Attention_Update output int16; Delta_Current_next output int16; Delta_Current_actual output int16; Current_Read local int16; Counter_Sample_Current local uint8; Current_Read_Average output int16; Delta_Current local int16; Reset_Filter output uint8; Current_Peak local int16; Delta_Current_previuos local int16; CounterVectorDownBwd_Read input uint16 size=13; CounterVectorUpFwd_Read input uint16 size=13; CounterVectorDownBwd_Write output uint16 size=13; CounterVectorUpFwd_Write output uint16 size=13; BitMaskIndex local uint8; BitPosition local uint8; UpdateTrh local uint8; CounterVectorDownFwd_Read input uint16 size=13; CounterVectorUpBwd_Read input uint16 size=13; CounterVectorDownFwd_Write output uint16 size=13; CounterVectorUpBwd_Write output uint16 size=13; firstsegment local double; Index_peak_time local uint8; Vbatt_Old local uint16; APSA_Delay local uint8; Cmd_Motor_Lift_Old local double
  data ResetCounter settings: description=$TL$ type=UInt8; date=20160120T160726; $TL$
  data ResetCounter settings: description=$TL$ type=UInt8; date=20160120T160726; $TL$
  data ResetCounter settings: description=$TL$ type=UInt8; date=20160120T160726; $TL$
  data ResetCounter settings: description=$TL$ type=UInt8; date=20160120T160726; $TL$
  data EERAM_Current_Map_Forward_Read settings: description=$TL$ date=20150907T181136; inheritscaling=1; $TL$
  data EERAM_Current_Map_Backward_Read settings: description=$TL$ date=20150916T160947; inheritscaling=1; $TL$
  data EERAM_Threshold_Attention_Forward settings: description=$TL$ date=20151006T184815; inheritscaling=1; $TL$
  data EERAM_Threshold_Attention_Backward settings: description=$TL$ date=20150916T161017; inheritscaling=1; $TL$
  data EERAM_Threshold_Antipinch_Forward settings: description=$TL$ date=20150916T161021; inheritscaling=1; $TL$
  data EERAM_Threshold_Antipinch_Backward settings: description=$TL$ variable=EERAM_Threshold_Antipinch_Backward; date=20151130T091528; inheritscaling=1; $TL$
  data Check_Antipinch settings: description=$TL$ date=20150916T161025; inheritscaling=1; $TL$
  data Cmd_Motor settings: description=$TL$ date=20150916T161032; inheritscaling=1; $TL$
  data Write_Map settings: description=$TL$ date=20150916T161037; inheritscaling=1; $TL$
  data Lenght_Motor_Stroke settings: description=$TL$ date=20150916T161040; inheritscaling=1; $TL$
  data Cmd_Motor_Lift settings: description=$TL$ type=UInt8; date=20160304T135854; $TL$
  data Hall_Counter_Forward settings: description=$TL$ date=20150916T161049; inheritscaling=1; $TL$
  data Hall_Counter_Backward settings: description=$TL$ date=20151001T094053; inheritscaling=1; $TL$
  data Current settings: description=$TL$ date=20150916T161056; inheritscaling=1; $TL$
  data Enable_APSA settings: description=$TL$ date=20150916T161100; inheritscaling=1; $TL$
  data Vbatt settings: description=$TL$ type=Int16; date=20160301T153029; $TL$
  data Lenght_Segment settings: description=$TL$ type=UInt8; date=20150916T160736; $TL$
  data EERAM_Current_Map_Forward_Write settings: description=$TL$ variable=EERAM_Current_Map_Forward; date=20151013T111909; $TL$
  data EERAM_Current_Map_Backward_Write settings: description=$TL$ variable=EERAM_Current_Map_Backward; date=20150916T161756; $TL$
  data Counter_Time settings: description=$TL$ type=UInt16; date=20150924T154526; $TL$
  data Average_EERAM_Current_Map settings: description=$TL$ type=Int16; date=20151130T091419; $TL$
  data Average_Current settings: description=$TL$ type=Int16; date=20160126T082918; $TL$
  data Mod settings: description=$TL$ type=UInt8; date=20150916T161012; $TL$
  data Segments_Cnt settings: description=$TL$ type=UInt8; date=20150916T162924; $TL$
  data Average_Difference settings: description=$TL$ type=Int16; date=20150924T160159; $TL$
  data Fail_Sens_Current settings: description=$TL$ name=$D; type=UInt8; scaling=VOID_SCALING; date=20151005T154451; $TL$
  data Cnt_Fail_Sens_Current settings: description=$TL$ type=UInt8; date=20151005T154406; $TL$
  data cnt_antipinch settings: description=$TL$ type=UInt16; date=20150916T160934; $TL$
  data DELTA_1 settings: description=$TL$ date=20150916T161104; inheritscaling=1; $TL$
  data DELTA_2 settings: description=$TL$ date=20150916T161118; inheritscaling=1; $TL$
  data DELTA_3 settings: description=$TL$ date=20150916T161122; inheritscaling=1; $TL$
  data DELTA_4 settings: description=$TL$ date=20150916T161125; inheritscaling=1; $TL$
  data Antipinch_Active settings: description=$TL$ name=$D; type=UInt8; scaling=VOID_SCALING; date=20151005T154728; $TL$
  data DELTA_5 settings: description=$TL$ date=20150916T161129; inheritscaling=1; $TL$
  data DELTA_6 settings: description=$TL$ date=20150916T161133; inheritscaling=1; $TL$
  data Index_vector settings: description=$TL$ type=UInt8; date=20150916T160942; $TL$
  data Threshold_AntiPinch_Update settings: description=$TL$ variable=Threshold_AntiPinch_Update; date=20151006T184415; $TL$
  data Threshold_Attention_Update settings: description=$TL$ variable=Threshold_Attention_Update; date=20151006T184411; $TL$
  data Delta_Current_next settings: description=$TL$ type=Int16; date=20151006T150218; $TL$
  data Delta_Current_actual settings: description=$TL$ type=Int16; date=20151006T150226; $TL$
  data Current_Read settings: description=$TL$ type=Int16; date=20151006T164240; $TL$
  data Counter_Sample_Current settings: description=$TL$ type=UInt8; date=20151007T121221; $TL$
  data Current_Read_Average settings: description=$TL$ type=Int16; date=20151007T121131; $TL$
  data Delta_Current settings: description=$TL$ type=Int16; date=20151130T091209; $TL$
  data Reset_Filter settings: description=$TL$ type=UInt8; date=20151123T113420; $TL$
  data Current_Peak settings: description=$TL$ type=Int16; date=20151209T104506; $TL$
  data Delta_Current_previuos settings: description=$TL$ type=Int16; date=20160118T180214; $TL$
  data CounterVectorDownBwd_Read settings: description=$TL$ variable=EERAM_CounterVectorDownBwd; date=20160120T154111; $TL$
  data CounterVectorUpFwd_Read settings: description=$TL$ variable=EERAM_CounterVectorUpFwd; date=20160120T154116; $TL$
  data CounterVectorDownBwd_Write settings: description=$TL$ variable=EERAM_CounterVectorDownBwd; date=20160120T154111; $TL$
  data CounterVectorUpFwd_Write settings: description=$TL$ variable=EERAM_CounterVectorUpFwd; date=20160120T154116; $TL$
  data BitMaskIndex settings: description=$TL$ type=UInt8; date=20160118T175958; $TL$
  data BitPosition settings: description=$TL$ type=UInt8; date=20160118T175958; $TL$
  data UpdateTrh settings: description=$TL$ type=UInt8; date=20160118T180001; $TL$
  data CounterVectorDownFwd_Read settings: description=$TL$ variable=EERAM_CounterVectorDownFwd; date=20160120T154210; $TL$
  data CounterVectorUpBwd_Read settings: description=$TL$ variable=EERAM_CounterVectorUpBwd; date=20160120T154230; $TL$
  data CounterVectorDownFwd_Write settings: description=$TL$ variable=EERAM_CounterVectorDownFwd; date=20160120T154221; $TL$
  data CounterVectorUpBwd_Write settings: description=$TL$ variable=EERAM_CounterVectorUpBwd; date=20160120T154232; $TL$
  data firstsegment settings: description=$TL$ type=UInt8; date=20160126T144809; $TL$
  data Index_peak_time settings: description=$TL$ type=UInt8; date=20160201T161907; $TL$
  data Vbatt_Old settings: description=$TL$ type=Int16; date=20160301T153013; $TL$
  data APSA_Delay settings: description=$TL$ type=UInt8; date=20160301T155543; $TL$
  data Cmd_Motor_Lift_Old settings: description=$TL$ type=UInt8; date=20160304T135857; $TL$

== stateflow chart APSA/APSA_OUTPUT/Create_Signal_Map_Backward ==
  state Calculate_Lenght_Segment [function]
    (default) -> (junction 37) : {Mod=Lenght_Motor_Stroke%%MAX_NUM_ELEMENT;}
    (junction 37) -> (junction 36) [order 1] : [Mod==0]
    (junction 37) -> (junction 38) [order 2]
    (junction 36) -> (junction 39) : {Lenght_Segment=Lenght_Motor_Stroke/MAX_NUM_ELEMENT;}
    (junction 38) -> (junction 41) : {Lenght_Segment=((Lenght_Motor_Stroke/MAX_NUM_ELEMENT)+1);}
    (junction 39) -> (junction 40)
    (junction 41) -> (junction 40)
    (junction 40) -> (junction 42)
  state WRITE_MAP_BACKWARD
    en:
    Index_vector=Hall_Counter_Backward/Lenght_Segment;
    Current_Read=0;
    Counter_Sample_Current=0;
    WRITE_MAP_BACKWARD -> (junction 54)
    (junction 54) -> (junction 55) [order 1] : [Hall_Counter_Backward>=((Index_vector*Lenght_Segment)+Lenght_Segment) && Index_vector<=MAX_NUM_ELEMENT-1]
    (junction 55) -> (junction 56) [order 1] : [Counter_Sample_Current==0 ||Current_Read==0 ]
    (junction 54) -> (junction 57) [order 2] : /*{Current_Read += Current;
        | Counter_Sample_Current++;}*/
    (junction 55) -> (junction 58) [order 2] : {Current_Read_Average = Current_Read/Counter_Sample_Current;}
    (junction 56) -> (junction 59) : {Current_Read_Average=Current;}
    (junction 58) -> (junction 57) : {EERAM_Current_Map_Backward_Write[Index_vector]=Current_Read_Average;
        | Mappa=EERAM_Current_Map_Backward_Write[Index_vector];
        | Current_Read=0;
        | Counter_Sample_Current=0;
        |  Index_vector++;}
    (junction 59) -> (junction 58)
    (junction 57) -> (junction 60)
  (default) -> WRITE_MAP_BACKWARD : {Calculate_Lenght_Segment();}
  data: EERAM_Current_Map_Backward_Write output size=100; Lenght_Motor_Stroke input; index_vector local double; mod local double; Lenght_Segment local uint8; Mod local double; Cmd_Motor input; Current input; Hall_Counter_Backward input; Counter_Sample_Current local double; Current_Read local double; Current_Read_Average local double; Index_vector output double; Mappa output double
  data EERAM_Current_Map_Backward_Write settings: description=$TL$ variable=EERAM_Current_Map_Backward; date=20150916T162456; $TL$
  data Lenght_Motor_Stroke settings: description=$TL$ date=20150916T162504; inheritscaling=1; $TL$
  data index_vector settings: description=$TL$ type=UInt8; date=20150916T161828; $TL$
  data mod settings: description=$TL$ type=UInt8; date=20150916T161846; $TL$
  data Lenght_Segment settings: description=$TL$ type=UInt8; date=20150916T161810; $TL$
  data Mod settings: description=$TL$ type=UInt8; date=20150916T161834; $TL$
  data Cmd_Motor settings: description=$TL$ date=20150916T162507; inheritscaling=1; $TL$

== stateflow chart APSA/APSA_OUTPUT/Create_Signal_Map_Forward ==
  state Calculate_Lenght_Segment [function]
    (default) -> (junction 38) : {Mod=Lenght_Motor_Stroke%%MAX_NUM_ELEMENT;}
    (junction 38) -> (junction 37) [order 1] : [Mod==0]
    (junction 38) -> (junction 39) [order 2]
    (junction 37) -> (junction 40) : {Lenght_Segment=Lenght_Motor_Stroke/MAX_NUM_ELEMENT;}
    (junction 39) -> (junction 42) : {Lenght_Segment=((Lenght_Motor_Stroke/MAX_NUM_ELEMENT)+1);}
    (junction 40) -> (junction 41)
    (junction 42) -> (junction 41)
    (junction 41) -> (junction 43)
  state CREATE_SIGN
    CREATE_SIGN -> (junction 15) : {Calculate_Lenght_Segment();
        | mod=Hall_Counter %% Lenght_Segment;}
    (junction 15) -> (junction 16) [order 1] : [mod==0 && Hall_Counter<=Lenght_Motor_Stroke && Hall_Counter!=0 && Cmd_Motor ==APSA_CMD_FORWARD]
    (junction 15) -> (junction 19) [order 2]
    (junction 16) -> (junction 20) : {index_vector= ((Hall_Counter/Lenght_Segment)-1);
        | Map_Signal=EERAM_Current_Map_Forward_Write[index_vector];}
    (junction 20) -> (junction 19)
    (junction 19) -> (junction 23)
  data: EERAM_Current_Map_Forward_Write input size=100; Hall_Counter input; Lenght_Motor_Stroke input; index_vector local double; Map_Signal output double; mod local double; Lenght_Segment local uint8; Mod local double; Cmd_Motor input
  data EERAM_Current_Map_Forward_Write settings: description=$TL$ variable=EERAM_Current_Map_Forward; date=20150916T162634; $TL$
  data Hall_Counter settings: description=$TL$ date=20150916T162641; inheritscaling=1; $TL$
  data Lenght_Motor_Stroke settings: description=$TL$ date=20150916T162722; inheritscaling=1; $TL$
  data index_vector settings: description=$TL$ type=UInt8; date=20150916T162544; $TL$
  data Map_Signal settings: description=$TL$ type=UInt16; date=20151005T154412; $TL$
  data mod settings: description=$TL$ type=UInt8; date=20150916T162610; $TL$
  data Lenght_Segment settings: description=$TL$ type=UInt8; date=20150916T162526; $TL$
  data Mod settings: description=$TL$ type=UInt8; date=20150916T162536; $TL$
  data Cmd_Motor settings: description=$TL$ date=20150916T162650; inheritscaling=1; $TL$

== stateflow chart APSA/Subsystem/APSA/FILTER8samples1/Average_mobile_Filter_8samp ==
  state AVERAGE
    AVERAGE -> (junction 102) [order 1] : {sum_weights=1;
        | sum_samples=0;}
    (junction 102) -> (junction 103) : {index_vector_filter=0;}
    (junction 105) -> (junction 111) : {circular_buffer[index_vector_filter] = circular_buffer[index_vector_filter+1];
        | sum_samples += circular_buffer[index_vector_filter];}
    (junction 103) -> (junction 105) [order 1] : [index_vector_filter < SIZE_FILTER-1]
    (junction 111) -> (junction 142) [order 1] : [circular_buffer[index_vector_filter] !=0]
        | {sum_weights += 1;}
    (junction 111) -> (junction 142) [order 2]
    (junction 107) -> (junction 103) : {index_vector_filter+=1;}
    (junction 103) -> (junction 151) [order 2] : {circular_buffer[index_vector_filter] = Current_AD;
        | sum_samples += circular_buffer[index_vector_filter] ;
        | average_filter = sum_samples/sum_weights;}
    (junction 142) -> (junction 107)
  (default) -> AVERAGE : {circular_buffer=0;}
  AVERAGE -> AVERAGE [order 1] : [Reset_Filter == 1]
      | {circular_buffer=0;}
  data: Current_AD input uint16; average_filter output int16; circular_buffer local uint16 size=8; index_vector_filter local uint8; sum_samples local int16; sum_weights local int16; Reset_Filter input uint8
  data Current_AD settings: description=$TL$ type=UInt16; date=20151130T092758; $TL$
  data average_filter settings: description=$TL$ type=Int16; date=20151203T091526; $TL$
  data circular_buffer settings: description=$TL$ name=circular_buffer; type=Int16; date=20151203T091754; $TL$
  data index_vector_filter settings: description=$TL$ type=UInt8; date=20151012T114749; $TL$
  data sum_samples settings: description=$TL$ type=Int16; date=20151203T091517; $TL$
  data sum_weights settings: description=$TL$ type=Int16; date=20151203T091543; $TL$
